simulink model "sys_360"  (R2024a)
settings: Solver=ode3  StartTime=0.0  StopTime=T_end  FixedStep=Ts  RelTol=1e-3
values from neighbouring files (symbols this model uses):
  Ts = 0.0005    [main_COProjection.m]    (also in main_Oblique.m)
  tt = 1    [main_COProjection.m]    (also in main_Oblique.m)
libraries: spspowerguiLib x1
settings Model: Creator=WAJ  LastModifiedBy=WAJ
settings SolverCC: AlgebraicLoopSolver=TrustRegion
settings DataIOCC: ReturnWorkspaceOutputs=off
settings DebuggingCC: UnconnectedInputMsg=warning  UnconnectedOutputMsg=warning  UnconnectedLineMsg=warning
settings ModelReferenceCC: EnableRefExpFcnMdlSchedulingChecks=on
settings RTWCC: GPUComputeCapability=3.5

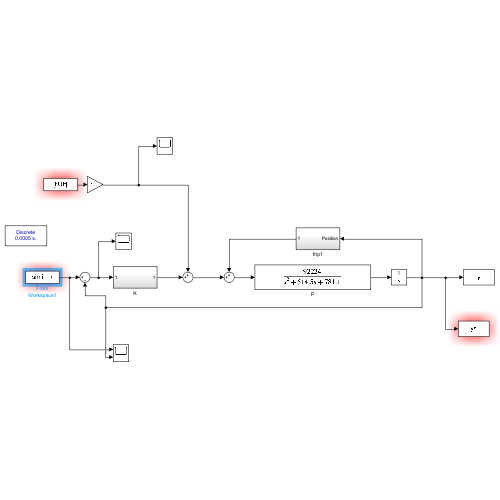
[thumbnail: Simulink's stored preview of the top-level diagram]
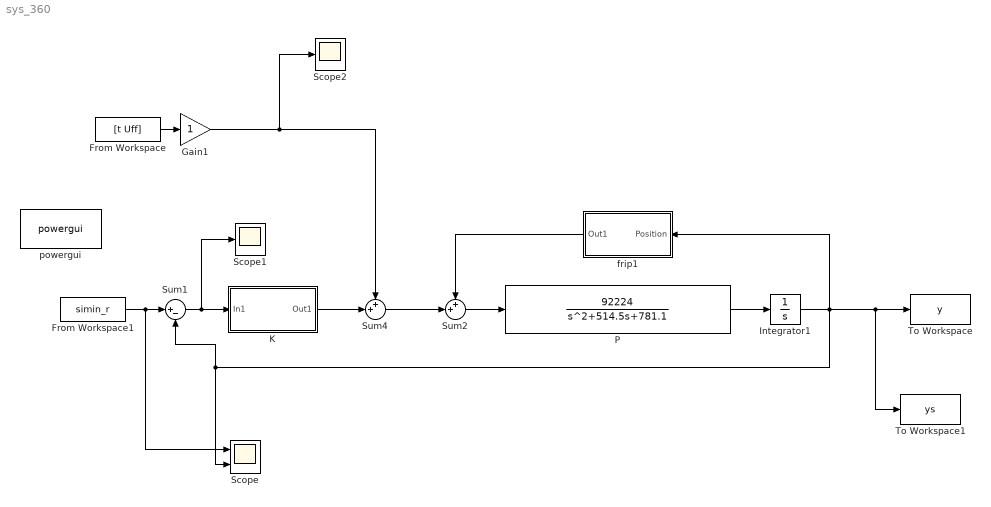
== system sys_360 ==
  From Workspace : FromWorkspace  VariableName=[t Uff]  SampleTime=Ts
  From Workspace1 : FromWorkspace  VariableName=simin_r
  Gain1 : Gain
  Integrator1 : Integrator
  K : Subsystem
  P : TransferFcn  Numerator=[92224]  Denominator=[1 514.5 781.1]
  Scope : Scope  NumInputPorts=2
  Scope1 : Scope
  Scope2 : Scope
  Sum1 : Sum  Inputs=|+-
  Sum2 : Sum  Inputs=++|
  Sum4 : Sum  Inputs=++|
  To Workspace : ToWorkspace  VariableName=y  SampleTime=Ts
  To Workspace1 : ToWorkspace  VariableName=ys  SampleTime=Ts*tt
  frip1 : Subsystem
  powergui : spspowerguiLib/powergui  Priority=1  SimulationMode=Discrete  SampleTime=0.0005  frequency=60  Iterations=50  frequencyindice=60  Pbase=100e6  ErrMax=1e-4  UnitsV=kV  UnitsW=MW  buscounter=0  FunctionMessages=off  echomessages=off  EnableUseOfTLC=off  CurrentSourceSwitches=off  DisableSnubberDevices=off  DisableRonSwitches=off  DisableVfSwitches=off  DisplayEquations=off  AutomaticDiscreteSolvers=off  SolverType=Tustin/Backward Euler (TBE)  Interpol=off  ExternalGateDelay=off  methode=off  Ts=100  x0status=blocks  SPID=on  SwTol=0  HookPort=off  NonlinearTolerance=1e-4  nMaxIteration=100  ContinueOnMaxIteration=off  RestoreLinks=warning  ResistiveCurrentMeasurement=off  Frange=[0:2:500]  Ylog=off  Xlog=on  ShowGrid=off  save=off  variable=ZData  structure=e_js  ZoomFFT=off  StartTime=1  cycles=8  DisplayStyle=1  fundamental=1  FreqAxis=off  MaxFrequency=10  frequencyindicesteady=1  RmsSteady=1  display=off
  wires:
  K/1(Out1) -> Sum4/2
  Sum1/1 -> K/1(In1), Scope1/1
  Sum4/1 -> Sum2/2
  Sum2/1 -> P/1
  From Workspace1/1 -> Scope/1, Sum1/1
  P/1 -> Integrator1/1
  Integrator1/1 -> frip1/1(Position), To Workspace1/1, To Workspace/1, Sum1/2, Scope/2
  From Workspace/1 -> Gain1/1
  Gain1/1 -> Scope2/1, Sum4/1
  frip1/1(Out1) -> Sum2/1

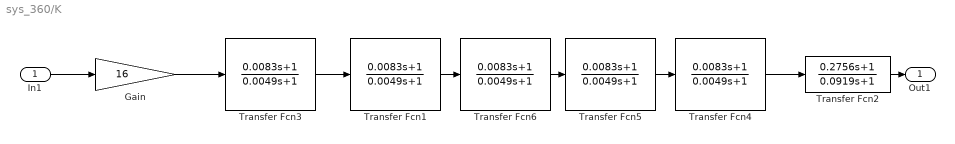
== system sys_360/K ==
  In1 : Inport
  Gain : Gain  Gain=16
  Transfer Fcn{1,3..6} (5 alike) : TransferFcn  Numerator=[0.0083 1]  Denominator=[0.0049 1]
  Transfer Fcn2 : TransferFcn  Numerator=[0.2756 1]  Denominator=[0.0919 1]
  Out1 : Outport  VectorParamsAs1DForOutWhenUnconnected=off
  wires:
  In1/1 -> Gain/1
  Gain/1 -> Transfer Fcn3/1
  Transfer Fcn3/1 -> Transfer Fcn1/1
  Transfer Fcn2/1 -> Out1/1
  Transfer Fcn1/1 -> Transfer Fcn6/1
  Transfer Fcn6/1 -> Transfer Fcn5/1
  Transfer Fcn5/1 -> Transfer Fcn4/1
  Transfer Fcn4/1 -> Transfer Fcn2/1

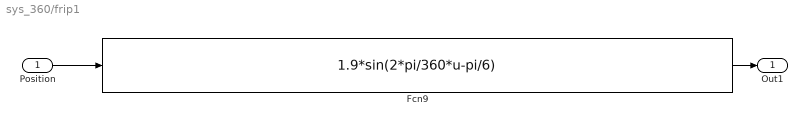
== system sys_360/frip1 ==
  Position : Inport
  Fcn9 : Fcn  Expr=1.9*sin(2*pi/360*u-pi/6)
  Out1 : Outport  VectorParamsAs1DForOutWhenUnconnected=off
  wires:
  Position/1 -> Fcn9/1
  Fcn9/1 -> Out1/1
